simulink model "Simulation_manual"  (R2017a)
settings: Solver=VariableStepAuto  StartTime=0.0  StopTime=150  RelTol=1e-3  EnableMultiTasking=on
InitFcn:
  | load('Parameters.mat');
undefined symbols (not defined in the file or in its folder): A_AC_LONG_SS, B_AC_LONG_SS, C_AC_LONG_SS, D_AC_LONG_SS, int_time, RW_Alt, trim_control_hi, trim_state_hi, trim_thrust_hi, velocity
libraries: aerolibfltsims x2, vrlib x1
settings Model: Creator=Y Nie  LastModifiedBy=aelabuser
settings DataIOCC: SaveFormat=Array  SaveOutput=off  SignalLogging=off  DSMLogging=off  TimeSaveName=SimTime
settings OptimizationCC: ExpressionDepthLimit=2147483647  LifeSpan=inf
settings DebuggingCC: UnderspecifiedInitializationDetection=Classic  MergeDetectMultiDrivingBlocksExec=none  FcnCallInpInsideContextMsg=warning  StateNameClashWarn=warning  SFUnexpectedBacktrackingDiag=warning  SFNoUnconditionalDefaultTransitionDiag=warning  SFExecutionAtInitializationDiag=none
settings HardwareCC: ProdBitPerPointer=32  ProdBitPerSizeT=32  ProdBitPerPtrDiffT=32  ProdLargestAtomicFloat=None  ProdIntDivRoundTo=Undefined  ProdEndianess=Unspecified  ProdWordSize=32  ProdHWDeviceType=32-bit Generic
settings ModelReferenceCC: PropagateSignalLabelsOutOfModel=off
settings GRTTargetCC: TargetLangStandard=C89/C90 (ANSI)  GeneratePreprocessorConditionals=Disable all  CombineOutputUpdateFcns=off  GRTInterface=on
settings ConfigComp: CovMetricSettings=dw  CovHtmlReporting=on  CovSaveCumulativeToWorkspaceVar=on  CovSaveSingleToWorkspaceVar=on  CovExternalEMLEnable=off

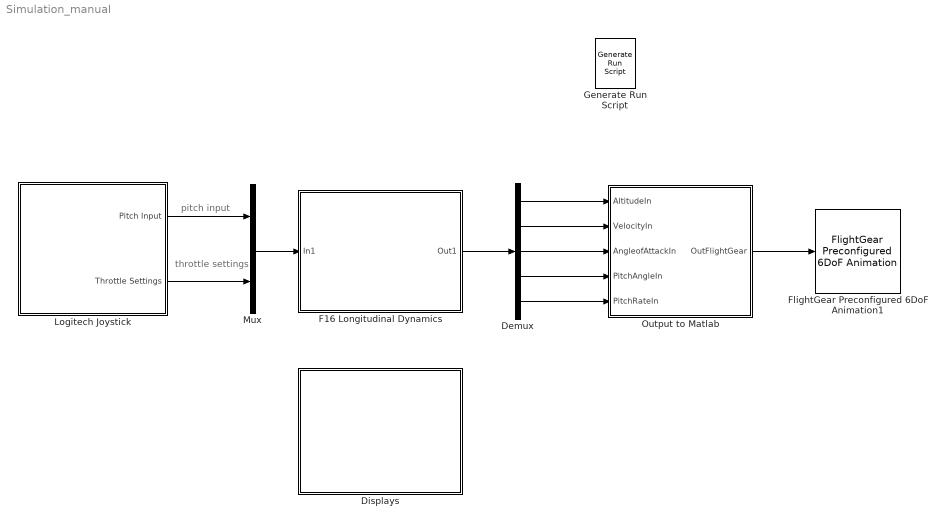
== system Simulation_manual ==
  note: throttle settings
  note: pitch input
  Demux : Demux  Outputs=[1 1 1 1 1]
  Displays : Subsystem
      mask Display: image('f16display.jpg');
  F16 Longitudinal Dynamics : Subsystem
      mask Display: image(imread('f16thumb.jpg'))
  FlightGear Preconfigured 6DoF Animation1 : aerolibfltsims/FlightGear Preconfigured 6DoF Animation  xFlightGearVersion=v2016.3  DestinationIpAddress=146.169.191.46  DestinationPort=5502  SampleTime=0.005
      settings: SourceProductName=Aerospace Blockset
  Generate Run Script : aerolibfltsims/Generate Run Script  OutputFileName=runfg.bat  FlightGearBaseDirectory=F:\Program Files\FlightGear 3.4.0  GeometryModelName=fokker100  DestinationPort=5502  OriginAddress=127.0.0.1  OriginPort=5505  LocalAddress=127.0.0.1  AirportId=KSFO  RunwayId=10L  InitialAltitude=5000  InitialHeading=113  OffsetDistance=4.72  OffsetAzimuth=0  GenerateFile=off  Architecture=Default  dataFlow=Send
  Logitech Joystick : Subsystem
      mask Display: image(imread('LogitechJoystick.jpg'))
  Mux : Mux  Inputs=2
  Output to Matlab : Subsystem
  wires:
  Mux/1 -> F16 Longitudinal Dynamics/1(In1)
  Demux/2 -> Output to Matlab/2(VelocityIn)
  F16 Longitudinal Dynamics/1(Out1) -> Demux/1
  Demux/5 -> Output to Matlab/5(PitchRateIn)
  Demux/1 -> Output to Matlab/1(AltitudeIn)
  Demux/3 -> Output to Matlab/3(AngleofAttackIn)
  Demux/4 -> Output to Matlab/4(PitchAngleIn)
  Output to Matlab/1(OutFlightGear) -> FlightGear Preconfigured 6DoF Animation1/1
  Logitech Joystick/1(Pitch Input) -> Mux/1
  Logitech Joystick/2(Throttle Settings) -> Mux/2

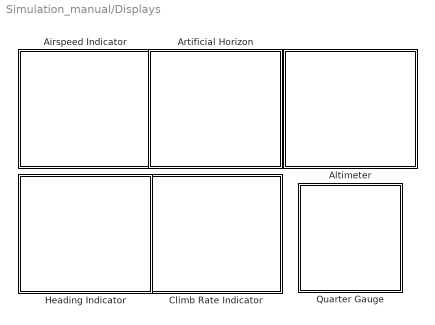
== system Simulation_manual/Displays ==
  Airspeed Indicator : Subsystem  DialogController=aeroblksHMICreateDDGDialog  IsWebBlock=on  mask(MWDashboardBlock){webBlockId=b3892bee-502b-44ef-811e-2493f59221ea, webBlockType=airspeedindicator, ShowLibInBrowser=on, ShowInitialText=on, HMISrcModelName=Simulation_manual}
      mask prompts: webBlockId "WebBlock Id"; webBlockType "WebBlock Type"; HMISrcModelName "Source Model"
      mask Help: eval('asbhmihelp(''airspeedindicator'')');
      mask Display:
      | if strcmp(get_param(bdroot(gcb),'BlockDiagramType'), 'library')
      |  image([(matlabroot) '/toolbox/aeroblks/aeroblks/hmi/icons/AirspeedIndicatorIcon.svg'])
      | end
  Altimeter : Subsystem  DialogController=aeroblksHMICreateDDGDialog  IsWebBlock=on  mask(MWDashboardBlock){webBlockId=a0b9298c-5785-4919-b7f8-c7cccb17a8c9, webBlockType=altimeter, ShowLibInBrowser=on, ShowInitialText=on, HMISrcModelName=Simulation_manual}
      mask prompts: webBlockId "WebBlock Id"; webBlockType "WebBlock Type"; HMISrcModelName "Source Model"
      mask Help: eval('asbhmihelp(''altimeter'')');
      mask Display:
      | if strcmp(get_param(bdroot(gcb),'BlockDiagramType'), 'library')
      |  image([(matlabroot) '/toolbox/aeroblks/aeroblks/hmi/icons/AltimeterIcon.svg'])
      | end
  Artificial Horizon : Subsystem  DialogController=aeroblksHMICreateDDGDialog  IsWebBlock=on  mask(MWDashboardBlock){webBlockId=7012071a-1ac7-465e-b6e9-c94febfd6ad2, webBlockType=artificialhorizon, ShowLibInBrowser=on, ShowInitialText=on, HMISrcModelName=Simulation_manual}
      mask prompts: webBlockId "WebBlock Id"; webBlockType "WebBlock Type"; HMISrcModelName "Source Model"
      mask Help: eval('asbhmihelp(''artificialhorizon'')');
      mask Display:
      | if strcmp(get_param(bdroot(gcb),'BlockDiagramType'), 'library')
      |  image([(matlabroot) '/toolbox/aeroblks/aeroblks/hmi/icons/ArtificialHorizonIcon.svg'])
      | end
  Climb Rate Indicator : Subsystem  DialogController=aeroblksHMICreateDDGDialog  IsWebBlock=on  mask(MWDashboardBlock){webBlockId=c36a9585-9208-4b6d-804b-ff501efecac2, webBlockType=climbindicator, ShowLibInBrowser=on, ShowInitialText=on, HMISrcModelName=Simulation_manual}
      mask prompts: webBlockId "WebBlock Id"; webBlockType "WebBlock Type"; HMISrcModelName "Source Model"
      mask Help: eval('asbhmihelp(''climbindicator'')');
      mask Display:
      | if strcmp(get_param(bdroot(gcb),'BlockDiagramType'), 'library')
      |  image([(matlabroot) '/toolbox/aeroblks/aeroblks/hmi/icons/ClimbIndicatorIcon.svg'])
      | end
  Heading Indicator : Subsystem  DialogController=aeroblksHMICreateDDGDialog  IsWebBlock=on  mask(MWDashboardBlock){webBlockId=da6ed19f-560c-41e9-974d-f470a470f1c0, webBlockType=headingindicator, ShowLibInBrowser=on, ShowInitialText=on, HMISrcModelName=Simulation_manual}
      mask prompts: webBlockId "WebBlock Id"; webBlockType "WebBlock Type"; HMISrcModelName "Source Model"
      mask Help: eval('asbhmihelp(''headingindicator'')');
      mask Display:
      | if strcmp(get_param(bdroot(gcb),'BlockDiagramType'), 'library')
      |  image([(matlabroot) '/toolbox/aeroblks/aeroblks/hmi/icons/HeadingIndicatorIcon.svg'])
      | end
  Quarter Gauge : Subsystem  DialogController=hmiCreateDDGDialog  IsWebBlock=on  mask(MWDashboardBlock){webBlockId=35e0a69a-9614-4fa9-a19d-d944fb4c325d, webBlockType=ninetydegreegauge, ShowInLibBrowser=on, ShowInitialText=on, HMISrcModelName=Simulation_manual}
      mask prompts: webBlockId "WebBlock Id"; webBlockType "WebBlock Type"; HMISrcModelName "Source Model"
      mask help: SimulinkHMI:dialogs:NinetydegreeGaugeDialogDesc
      mask Help: helpview([docroot '/mapfiles/simulink.map'], 'hmi_quarter_gauge')
      mask Display:
      | if strcmp(get_param(bdroot(gcb),'BlockDiagramType'), 'library')
      |     image([(matlabroot) '/toolbox/simulink/hmi/icons/NinetyDegreeGauge.png']);
      | end

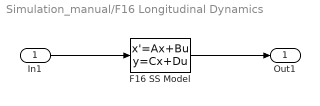
== system Simulation_manual/F16 Longitudinal Dynamics ==
  In1 : Inport
  F16 SS Model : StateSpace  A=A_AC_LONG_SS  B=B_AC_LONG_SS  C=C_AC_LONG_SS  D=D_AC_LONG_SS  X0=0
  Out1 : Outport
  wires:
  In1/1 -> F16 SS Model/1
  F16 SS Model/1 -> Out1/1

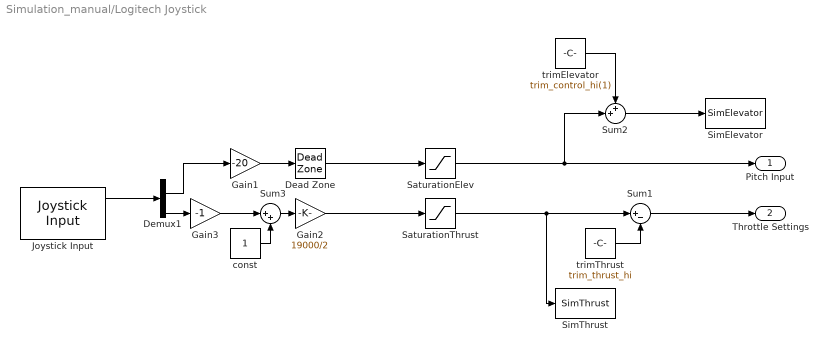
== system Simulation_manual/Logitech Joystick ==
  Dead Zone : DeadZone  LowerValue=-1  UpperValue=1  SaturateOnIntegerOverflow=on
  Demux1 : Demux
  Gain1 : Gain  Gain=-20
  Gain2 : Gain  Gain=19000/2
  Gain3 : Gain  Gain=-1
  Joystick Input : vrlib/Joystick Input  joyid=1  adjustports=on  forcefeed=off
      settings: SourceProductBaseCode=VR
  SaturationElev : Saturate  UpperLimit=25-trim_control_hi(1)  LowerLimit=-25-trim_control_hi(1)
  SaturationThrust : Saturate  UpperLimit=19000  LowerLimit=1000
  SimElevator : ToWorkspace  VariableName=SimElevator  SampleTime=-1
  SimThrust : ToWorkspace  VariableName=SimThrust  SampleTime=-1
  Sum1 : Sum  Inputs=|+-
  Sum2 : Sum  Inputs=++|
  Sum3 : Sum  Inputs=|++
  const : Constant
  trimElevator : Constant  Value=trim_control_hi(1)
  trimThrust : Constant  Value=trim_thrust_hi
  Pitch Input : Outport
  Throttle Settings : Outport  Port=2
  wires:
  Demux1/2 -> Gain1/1
  Joystick Input/1 -> Demux1/1
  Demux1/4 -> Gain3/1
  Gain1/1 -> Dead Zone/1
  Gain3/1 -> Sum3/1
  SaturationThrust/1 -> SimThrust/1, Sum1/1
  const/1 -> Sum3/2
  Sum1/1 -> Throttle Settings/1
  Gain2/1 -> SaturationThrust/1
  trimThrust/1 -> Sum1/2
  Sum3/1 -> Gain2/1
  Dead Zone/1 -> SaturationElev/1
  trimElevator/1 -> Sum2/1
  Sum2/1 -> SimElevator/1
  SaturationElev/1 -> Sum2/2, Pitch Input/1

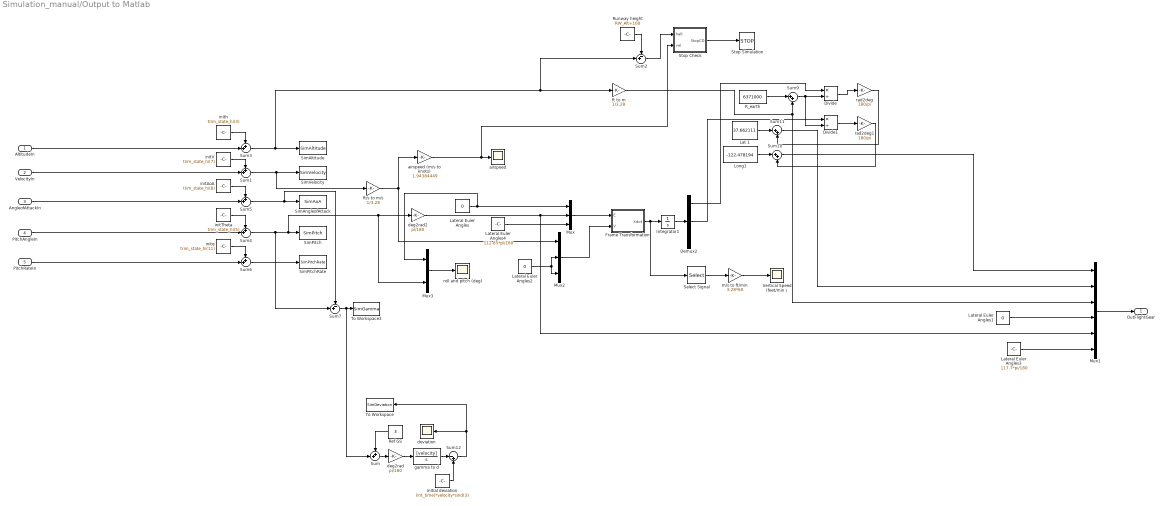
== system Simulation_manual/Output to Matlab ==
  AltitudeIn : Inport
  VelocityIn : Inport  Port=2
  AngleofAttackIn : Inport  Port=3
  PitchAngleIn : Inport  Port=4
  PitchRateIn : Inport  Port=5
  Demux2 : Demux  Outputs=3
  Divide : Product  Inputs=*/
  Divide1 : Product  Inputs=*/
  Frame Transformation : MATLAB Function  TreatAsAtomicUnit=on
  Initial deviation : Constant  Value=(int_time)*velocity*sind(3)
  Integrator1 : Integrator
  Lat 1 : Constant  Value=37.662111
  Lateral Euler Angles : Constant  Value=0
  Lateral Euler Angles1 : Constant  Value=0
  Lateral Euler Angles2 : Constant  Value=0
  Lateral Euler Angles3 : Constant  Value=117.7*pi/180
  Lateral Euler Angles4 : Constant  Value=112.85*pi/180
  Long1 : Constant  Value=-122.478194
  Mux : Mux  Inputs=3
  Mux1 : Mux  Inputs=6
  Mux2 : Mux  Inputs=3
  Mux3 : Mux  Inputs=2
  R_earth : Constant  Value=6371000
  Ref GS : Constant  Value=3
  Runway height : Constant  Value=RW_Alt+100
  "Select Signal " : Selector  InputPortWidth=3  IndexOptions=Index vector (dialog)  Indices=3  OutputSizes=1
  SimAltitude : ToWorkspace  VariableName=SimAltitude  SampleTime=-1
  SimAngleofAttack : ToWorkspace  VariableName=SimAoA  SampleTime=-1
  SimPitch : ToWorkspace  VariableName=SimPitch  SampleTime=-1
  SimPitchRate : ToWorkspace  VariableName=SimPitchRate  SampleTime=-1
  SimVelocity : ToWorkspace  VariableName=SimVelocity  SampleTime=-1
  Stop Check : MATLAB Function  TreatAsAtomicUnit=on
  Stop Simulation : Stop
  Sum{,1,3..6} (6 alike) : Sum  Inputs=++|
  Sum10 : Sum  Inputs=|++
  Sum11 : Sum  Inputs=|++
  Sum12 : Sum  Inputs=|-+
  Sum2 : Sum  Inputs=-+|
  Sum7 : Sum  Inputs=-+|
  Sum9 : Sum  Inputs=|++
  To Workspace : ToWorkspace  VariableName=SimDeviation  SampleTime=-1
  To Workspace3 : ToWorkspace  VariableName=SimGamma  SampleTime=-1
  Vertical Speed (feet/min） : Scope
  "airspeed " : Scope
  airspeed (m/s to knots) : Gain  Gain=1.94384449
  deg2rad : Gain  Gain=pi/180
  "deg2rad2 " : Gain  Gain=pi/180
  deviation : Scope
  ft to m : Gain  Gain=1/3.28
  ft/s to m/s : Gain  Gain=1/3.28
  gamma to d : TransferFcn  Numerator=[velocity]  Denominator=[1 0]
  initAoA : Constant  Value=trim_state_hi(8)
  initTheta : Constant  Value=trim_state_hi(5)
  initV : Constant  Value=trim_state_hi(7)
  inith : Constant  Value=trim_state_hi(3)
  initq : Constant  Value=trim_state_hi(11)
  "m/s to ft/min " : Gain  Gain=3.28*60
  rad2deg : Gain  Gain=180/pi
  rad2deg1 : Gain  Gain=180/pi
  roll and pitch (deg) : Scope
  OutFlightGear : Outport
  wires:
  inith/1 -> Sum3/1
  Sum5/1 -> Sum7/1, SimAngleofAttack/1
  Sum6/1 -> SimPitchRate/1
  PitchRateIn/1 -> Sum6/2
  initAoA/1 -> Sum5/1
  PitchAngleIn/1 -> Sum4/2
  Sum1/1 -> SimVelocity/1, ft/s to m/s/1
  initV/1 -> Sum1/1
  initTheta/1 -> Sum4/1
  AltitudeIn/1 -> Sum3/2
  AngleofAttackIn/1 -> Sum5/2
  VelocityIn/1 -> Sum1/2
  initq/1 -> Sum6/1
  Frame Transformation/1(Xdot) -> "Select Signal "/1, Integrator1/1
  Long1/1 -> Sum10/1
  Lateral Euler Angles3/1 -> Mux1/6
  Sum10/1 -> Mux1/1
  Integrator1/1 -> Demux2/1
  Sum9/1 -> Divide1/2, Divide/2
  Demux2/1 -> Divide/1
  ft to m/1 -> Sum9/2, Mux1/3
  Lat 1/1 -> Sum11/1
  Demux2/2 -> Divide1/1
  rad2deg/1 -> Sum11/2
  R_earth/1 -> Sum9/1
  Lateral Euler Angles2/1 -> Mux2/2, Mux2/3
  Lateral Euler Angles1/1 -> Mux1/4
  rad2deg1/1 -> Sum10/2
  Lateral Euler Angles4/1 -> Mux/3
  Sum4/1 -> Sum7/2, Mux3/2, "deg2rad2 "/1, SimPitch/1
  Lateral Euler Angles/1 -> Mux3/1, Mux/1
  Divide1/1 -> rad2deg1/1
  Mux2/1 -> Frame Transformation/2(V)
  Divide/1 -> rad2deg/1
  Sum3/1 -> Sum2/2, ft to m/1, SimAltitude/1
  Sum11/1 -> Mux1/2
  Mux/1 -> Frame Transformation/1(E)
  "deg2rad2 "/1 -> Mux1/5, Mux/2
  Mux1/1 -> OutFlightGear/1
  Runway height/1 -> Sum2/1
  Stop Check/1(StopCD) -> Stop Simulation/1
  Sum2/1 -> Stop Check/1(halt)
  ft/s to m/s/1 -> airspeed (m/s to knots)/1, Mux2/1
  airspeed (m/s to knots)/1 -> Stop Check/2(vel), "airspeed "/1
  Mux3/1 -> roll and pitch (deg)/1
  "Select Signal "/1 -> "m/s to ft/min "/1
  "m/s to ft/min "/1 -> Vertical Speed (feet/min）/1
  Sum/1 -> deg2rad/1
  Initial deviation/1 -> Sum12/2
  Sum12/1 -> deviation/1, To Workspace/1
  Ref GS/1 -> Sum/1
  Sum7/1 -> Sum/2, To Workspace3/1
  gamma to d/1 -> Sum12/1
  deg2rad/1 -> gamma to d/1

== system Simulation_manual/Displays/Airspeed Indicator ==

== system Simulation_manual/Displays/Altimeter ==

== system Simulation_manual/Displays/Artificial Horizon ==

== system Simulation_manual/Displays/Climb Rate Indicator ==

== system Simulation_manual/Displays/Heading Indicator ==

== system Simulation_manual/Displays/Quarter Gauge ==

== matlab function Simulation_manual/Output to Matlab/Stop Check ==
  data: halt input; StopCD output; vel input
function StopCD  = StopCheck(halt,vel)
%#codegen
if halt<0 
    StopCD=1;
elseif vel>240
    StopCD=1;
elseif vel<120
    StopCD=1;
else
    StopCD=0;
end

== matlab function Simulation_manual/Output to Matlab/Frame Transformation ==
  data: E input; Xdot output; V input
function Xdot = fcn(E,V)

%#codegen
% transformation from vertical ref. frame to body axes:
Rbv     = [1,  0,         0        ;
           0,  cos(E(1)), sin(E(1));
           0, -sin(E(1)), cos(E(1))]*...
          [cos(E(2)), 0, -sin(E(2));
           0,         1,  0        ;
           sin(E(2)), 0,  cos(E(2))]*...
          [cos(E(3)), sin(E(3)), 0 ;
          -sin(E(3)), cos(E(3)), 0 ;
           0,         0        , 1];


Xdot  = Rbv'*V;

Xdot(3)=-Xdot(3);
